simulink model "TP1"  (Simulink 9.0)
settings: Solver=VariableStepAuto  StartTime=0.0  StopTime=50  RelTol=1e-3
undefined symbols (not defined in the file): B, K, Ka, M, Ma, w
settings Model: Creator=BRIAN  LastModifiedBy=BRIAN
settings DataIOCC: SaveFormat=Dataset
settings OptimizationCC: UseFloatMulNetSlope=on  LifeSpan=auto
settings DebuggingCC: UnderspecifiedInitializationDetection=Simplified  MergeDetectMultiDrivingBlocksExec=error  SFUnexpectedBacktrackingDiag=error  SFNoUnconditionalDefaultTransitionDiag=error  SFExecutionAtInitializationDiag=warning
settings HardwareCC: ProdBitPerPointer=64  ProdBitPerSizeT=64  ProdBitPerPtrDiffT=64  ProdLargestAtomicFloat=Float  ProdIntDivRoundTo=Zero  ProdEndianess=LittleEndian  ProdWordSize=64  ProdHWDeviceType=Intel->x86-64 (Windows64)
settings ModelReferenceCC: PropagateSignalLabelsOutOfModel=on
settings CodeAppCC: StateflowObjectComments=off
settings GRTTargetCC: TargetLangStandard=C99 (ISO)
settings ConfigComp: CovMetricSettings=dwe  CovHtmlReporting=off  CovSaveCumulativeToWorkspaceVar=off  CovSaveSingleToWorkspaceVar=off  CovExternalEMLEnable=on

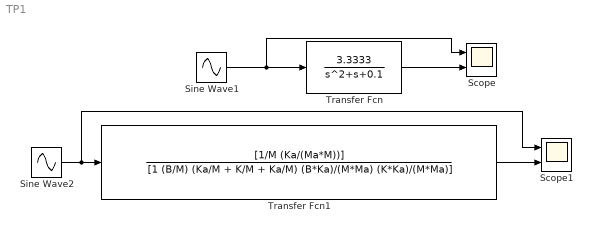
== system TP1 ==
  Scope : Scope  NumInputPorts=2
  Scope1 : Scope  NumInputPorts=2
  Sine Wave1 : Sin  Frequency=w  SampleTime=0
  Sine Wave2 : Sin  Frequency=w  SampleTime=0
  Transfer Fcn : TransferFcn  Numerator=[3.3333]  Denominator=[1 1 0.1]
  Transfer Fcn1 : TransferFcn  Numerator=[1/M (Ka/(Ma*M))]  Denominator=[1 (B/M) (Ka/M + K/M + Ka/M) (B*Ka)/(M*Ma) (K*Ka)/(M*Ma)]
  wires:
  Transfer Fcn/1 -> Scope/2
  Sine Wave1/1 -> Transfer Fcn/1, Scope/1
  Sine Wave2/1 -> Scope1/1, Transfer Fcn1/1
  Transfer Fcn1/1 -> Scope1/2
